simulink model "TrafficMoore"  (R2020b)
settings: Solver=VariableStepAuto  StartTime=0.0  StopTime=10.0  RelTol=1e-3
settings Model: Creator=DELL  LastModifiedBy=DELL

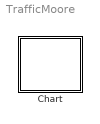
== system TrafficMoore ==
  Chart : Stateflow chart  TreatAsAtomicUnit=on

== stateflow chart TrafficMoore/Chart ==
  settings: stateMachineType=MOORE_MACHINE
